simulink model "bst_sl_model"  (R2015a)
settings: Solver=FixedStepDiscrete  StartTime=0.0  StopTime=T  FixedStep=Ts  RelTol=1e-3
libraries: simulink x1
settings Model: CovSFcnEnable=off  Creator=reiter  LastModifiedBy=reiter
settings DataIOCC: SignalLoggingSaveFormat=ModelDataLogs
settings DebuggingCC: UnderspecifiedInitializationDetection=Classic  MergeDetectMultiDrivingBlocksExec=none  SolverPrmCheckMsg=warning  MultiTaskDSMMsg=warning  MultiTaskCondExecSysMsg=none

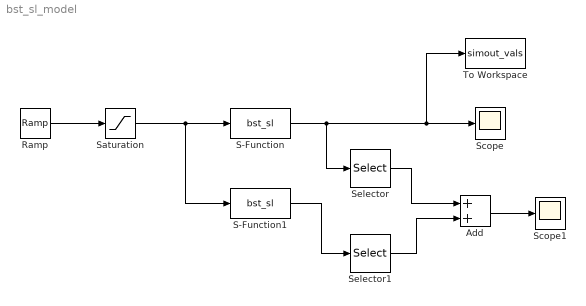
== system bst_sl_model ==
  Add : Sum
  Ramp : simulink/Sources/Ramp  slope=1  start=0  X0=0
  S-Function : S-Function  FunctionName=bst_sl  Parameters=spline, der_mask
  S-Function1 : S-Function  FunctionName=bst_sl  Parameters=spline, 0
  Saturation : Saturate  UpperLimit=1  LowerLimit=0
  Scope : Scope
  Scope1 : Scope
  Selector : Selector
  Selector1 : Selector
  To Workspace : ToWorkspace  VariableName=simout_vals  SampleTime=-1
  wires:
  Ramp/1 -> Saturation/1
  Saturation/1 -> S-Function1/1, S-Function/1
  S-Function/1 -> Selector/1, Scope/1, To Workspace/1
  Add/1 -> Scope1/1
  S-Function1/1 -> Selector1/1
  Selector/1 -> Add/1
  Selector1/1 -> Add/2
